simulink model "CMOS_Kernel_Memory_Sync"  (R2023b)
settings: Solver=VariableStepAuto  StartTime=0.0  StopTime=30000000  RelTol=1e-3
values from neighbouring files (symbols this model uses):
  AmountOfPixelsPerScanline = 400    [Kernel_Setup_Script.m]
  AmountOfRamBlocksScanlines = 5    [Kernel_Setup_Script.m]
  AmountOfRamBlocksScanlinesOffset = AmountOfRamBlocksScanlines - 1    (= 4)    [Kernel_Setup_Script.m]
  AmountOfScanlinePixels = 73700    [Kernel_Setup_Script.m]
  AmountOfScanlinePixelsOffset = AmountOfScanlinePixels - 1    (= 73699)    [Kernel_Setup_Script.m]
  AmountOfScanlines = 1100    [Kernel_Setup_Script.m]
  AmountOfScanlinesOffset = AmountOfScanlines - 1    (= 1099)    [Kernel_Setup_Script.m]
  AOPPK_Off = AmountOfPixelsPerScanline - 1    (= 399)    [Kernel_Setup_Script.m]
  AOPPS_Off = AmountOfPixelsPerScanline - 1    (= 399)    [Kernel_Setup_Script.m]
  FramePackOff_0 = FramePackOff_0 - ScanlineFifoCheck    [Kernel_Setup_Script.m]
  FramePackOff_1 = FramePackOff_1 - ScanlineFifoCheck    [Kernel_Setup_Script.m]
  FramePackOff_2 = FramePackOff_2 - ScanlineFifoCheck    [Kernel_Setup_Script.m]
  FramePackOff_3 = FramePackOff_3 - ScanlineFifoCheck    [Kernel_Setup_Script.m]
  FramePackOff_4 = FramePackOff_4 - ScanlineFifoCheck    [Kernel_Setup_Script.m]
  FramePackOff_5 = FramePackOff_5 - ScanlineFifoCheck    [Kernel_Setup_Script.m]
  KernelPackOff_0 = KernelPackOff_0 - KernelBitsPerRow    [Kernel_Setup_Script.m]
  KernelPackOff_1 = KernelPackOff_1 - KernelBitsPerRow    [Kernel_Setup_Script.m]
  KernelPackOff_2 = KernelPackOff_2 - KernelBitsPerRow    [Kernel_Setup_Script.m]
  KernelPackOff_3 = KernelPackOff_3 - KernelBitsPerRow    [Kernel_Setup_Script.m]
  Slice59DownTo48Top = (MsbOffset - (ScanlinePixelBitSizeController*1))    (= 59)    [Kernel_Setup_Script.m]
  Slice71DownTo60Top = (MsbOffset - (ScanlinePixelBitSizeController*0))    (= 71)    [Kernel_Setup_Script.m]
  TotalSectionsForFrames = AmountOfScanlines/AmountOfRamBlocksScanlines    (= 220)    [Kernel_Setup_Script.m]
  UltraRamRows = AmountOfPixelsPerScanline/ScanlineFifoCheck    [Kernel_Setup_Script.m]
  UltraRamRowsCeil = ceil(AmountOfPixelsPerScanline/ScanlineFifoCheck)    [Kernel_Setup_Script.m]
  UltraRamRowsKernel = AmountOfPixelsPerScanline/KernelBitsPerRow    (= 100)    [Kernel_Setup_Script.m]
  UltraRamRowsKernelCeil = ceil(AmountOfPixelsPerScanline/KernelBitsPerRow)    [Kernel_Setup_Script.m]
  UltraRamRowsMemorySectionOffset = UltraRamRowsCeil*AmountOfRamBlocksScanlines    [Kernel_Setup_Script.m]
  UltraRamRowsOffset = UltraRamRowsCeil - 1    [Kernel_Setup_Script.m]
undefined symbols (not defined in the file or in its folder): c, Down, sfvc784, Up, xck26
libraries: hdlBasic x4512, vmcUtilities x1
(part 11 of 39)

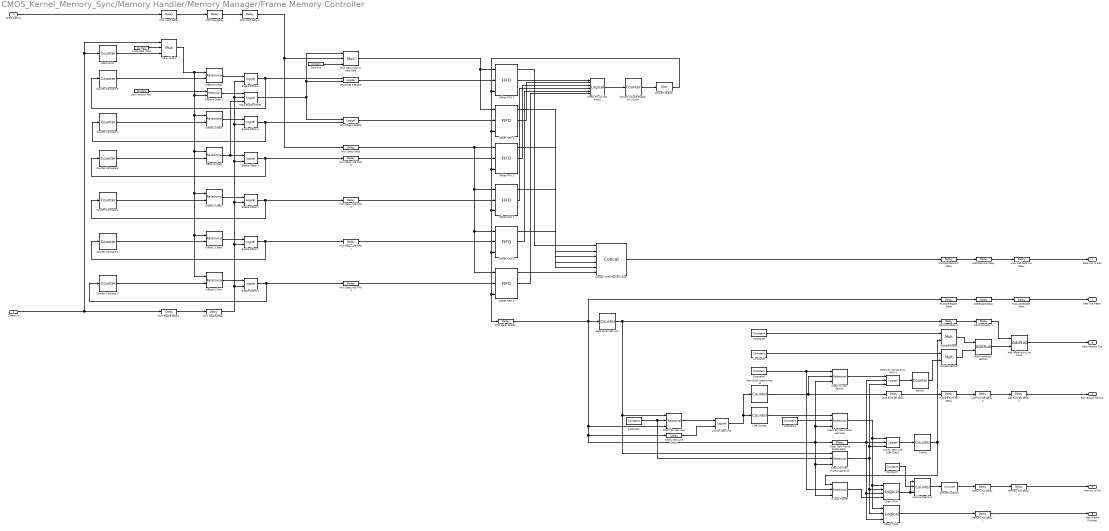
== system CMOS_Kernel_Memory_Sync/Memory Handler/Memory Manager/Frame Memory Controller ==
  12 Bit Data In : Inport
  Enable In : Inport  Port=2
  AND Input Delay : hdlBasic/Delay  rst=off  en=off  latency=1  reg_retiming=off  XmcBlockStatus=1  maskContainerNames=group1  block_type=delay  block_config=sysgen:Delay_config
  AND Input Delay2 : hdlBasic/Delay  rst=off  en=off  latency=1  reg_retiming=off  XmcBlockStatus=1  maskContainerNames=group1  block_type=delay  block_config=sysgen:Delay_config
  Add Data Out Delay : hdlBasic/Delay  rst=off  en=off  latency=1  reg_retiming=off  XmcBlockStatus=1  maskContainerNames=group1  block_type=delay  block_config=sysgen:Delay_config
  Add Enable Delay : hdlBasic/Delay  rst=off  en=off  latency=1  reg_retiming=off  XmcBlockStatus=1  maskContainerNames=group1  block_type=delay  block_config=sysgen:Delay_config
  Add Frame and Section : hdlBasic/AddSub  mode=Addition  use_carryin=off  use_carryout=off  en=off  latency=1  precision=Full  arith_type=Unsigned  n_bits=16  bin_pt=14  quantization=Truncate  overflow=Wrap  use_behavioral_HDL=off  hw_selection=Fabric  pipelined=off  XmcBlockStatus=1  maskContainerNames=tabcontainer1  block_type=addsub  block_config=sysgen:Addsub_config
  Add Line Delay 0 : hdlBasic/Delay  rst=off  en=off  latency=3  reg_retiming=off  XmcBlockStatus=1  maskContainerNames=group1  block_type=delay  block_config=sysgen:Delay_config
  Add Line Delay 1 : hdlBasic/Delay  rst=off  en=off  latency=1  reg_retiming=off  XmcBlockStatus=1  maskContainerNames=group1  block_type=delay  block_config=sysgen:Delay_config
  Add Offset with Line Count : hdlBasic/AddSub  mode=Addition  use_carryin=off  use_carryout=off  en=off  latency=1  precision=User Defined  arith_type=Unsigned  n_bits=ceil(log2(AmountOfScanlinePixels))  bin_pt=0  quantization=Truncate  overflow=Wrap  use_behavioral_HDL=off  hw_selection=Fabric  pipelined=off  XmcBlockStatus=1  maskContainerNames=tabcontainer1  block_type=addsub  block_config=sysgen:Addsub_config
  Add RAM Sel Delay 0 : hdlBasic/Delay  rst=off  en=off  latency=1  reg_retiming=off  XmcBlockStatus=1  maskContainerNames=group1  block_type=delay  block_config=sysgen:Delay_config
  Add RAM Sel Delay 1 : hdlBasic/Delay  rst=off  en=off  latency=1  reg_retiming=off  XmcBlockStatus=1  maskContainerNames=group1  block_type=delay  block_config=sysgen:Delay_config
  And RAM Sel Delay : hdlBasic/Delay  rst=off  en=off  latency=1  reg_retiming=off  XmcBlockStatus=1  maskContainerNames=group1  block_type=delay  block_config=sysgen:Delay_config
  And for New Line : hdlBasic/Logical  logical_function=AND  inputs=2  en=off  latency=1  precision=Full  arith_type=Unsigned  n_bits=16  bin_pt=0  align_bp=on  overflow=[]  quantization=[]  XmcBlockStatus=1  maskContainerNames=tabcontainer1  block_type=logical  block_config=sysgen:Logical_config
  And for New Line 1099 Check : hdlBasic/Logical  logical_function=AND  inputs=3  en=off  latency=1  precision=Full  arith_type=Unsigned  n_bits=16  bin_pt=0  align_bp=on  overflow=[]  quantization=[]  XmcBlockStatus=1  maskContainerNames=tabcontainer1  block_type=logical  block_config=sysgen:Logical_config
  Check For All Not Empty : hdlBasic/Logical  logical_function=NOR  inputs=6  en=off  latency=1  precision=Full  arith_type=Unsigned  n_bits=16  bin_pt=0  align_bp=on  overflow=[]  quantization=[]  XmcBlockStatus=1  maskContainerNames=tabcontainer1  block_type=logical  block_config=sysgen:Logical_config
  Check For New Frame Last Pixel : hdlBasic/Relational  mode=a=b  op_type=Bool  en=on  latency=1  XmcBlockStatus=1  maskContainerNames=tabcontainer1  block_type=relational  block_config=sysgen:Relational_config
  Check New Frame Enable Delay : hdlBasic/Delay  rst=off  en=off  latency=1  reg_retiming=off  XmcBlockStatus=1  maskContainerNames=group1  block_type=delay  block_config=sysgen:Delay_config
  Check New Line Delay : hdlBasic/Delay  rst=off  en=off  latency=1  reg_retiming=off  XmcBlockStatus=1  maskContainerNames=group1  block_type=delay  block_config=sysgen:Delay_config
  Check for New Frame Last Row : hdlBasic/Relational  mode=a=b  op_type=Bool  en=on  latency=1  XmcBlockStatus=1  maskContainerNames=tabcontainer1  block_type=relational  block_config=sysgen:Relational_config
  Check for last pixel on RAM 4 : hdlBasic/Logical  logical_function=AND  inputs=3  en=off  latency=1  precision=Full  arith_type=Unsigned  n_bits=16  bin_pt=0  align_bp=on  overflow=[]  quantization=[]  XmcBlockStatus=1  maskContainerNames=tabcontainer1  block_type=logical  block_config=sysgen:Logical_config
  Check for new Line : hdlBasic/Relational  mode=a=b  op_type=Bool  en=on  latency=1  XmcBlockStatus=1  maskContainerNames=tabcontainer1  block_type=relational  block_config=sysgen:Relational_config
  Check for new Section : hdlBasic/Relational  mode=a=b  op_type=Bool  en=on  latency=1  XmcBlockStatus=1  maskContainerNames=tabcontainer1  block_type=relational  block_config=sysgen:Relational_config
  Check if full : hdlBasic/Logical  logical_function=AND  inputs=4  en=off  latency=1  precision=Full  arith_type=Unsigned  n_bits=16  bin_pt=0  align_bp=on  overflow=[]  quantization=[]  XmcBlockStatus=1  maskContainerNames=tabcontainer1  block_type=logical  block_config=sysgen:Logical_config
  Check if full1 : hdlBasic/Logical  logical_function=AND  inputs=3  en=off  latency=1  precision=Full  arith_type=Unsigned  n_bits=16  bin_pt=0  align_bp=on  overflow=[]  quantization=[]  XmcBlockStatus=1  maskContainerNames=tabcontainer1  block_type=logical  block_config=sysgen:Logical_config
  Concat 72 Bit Packed Value : hdlBasic/Concat  num_inputs=ScanlineFifoCheck  XmcBlockStatus=1  maskContainerNames=group1  block_type=concat  block_config=sysgen:Concat_config
  Constant2 : hdlBasic/Constant  const=UltraRamRowsOffset  gui_display_data_type=Fixed-point  arith_type=Unsigned  n_bits=ceil(log2(UltraRamRows))  bin_pt=0  preci_type=Single  exp_width=8  frac_width=24  explicit_period=off  period=1  XmcBlockStatus=1  maskContainerNames=tabcontainer1  block_type=constant  block_config=sysgen:Constant_config
  Constant3 : hdlBasic/Constant  const=UltraRamRowsCeil  gui_display_data_type=Fixed-point  arith_type=Unsigned  n_bits=ceil(log2(UltraRamRowsCeil+1))  bin_pt=0  preci_type=Single  exp_width=8  frac_width=24  explicit_period=off  period=1  XmcBlockStatus=1  maskContainerNames=tabcontainer1  block_type=constant  block_config=sysgen:Constant_config
  Constant4 : hdlBasic/Constant  const=AmountOfScanlinesOffset  gui_display_data_type=Fixed-point  arith_type=Unsigned  n_bits=ceil(log2(AmountOfScanlines))  bin_pt=0  preci_type=Single  exp_width=8  frac_width=24  explicit_period=off  period=1  XmcBlockStatus=1  maskContainerNames=tabcontainer1  block_type=constant  block_config=sysgen:Constant_config
  Constant5 : hdlBasic/Constant  const=UltraRamRowsMemorySectionOffset  gui_display_data_type=Fixed-point  arith_type=Unsigned  n_bits=ceil(log2(UltraRamRowsMemorySectionOffset+1))  bin_pt=0  preci_type=Single  exp_width=8  frac_width=24  explicit_period=off  period=1  XmcBlockStatus=1  maskContainerNames=tabcontainer1  block_type=constant  block_config=sysgen:Constant_config
  Constant6 : hdlBasic/Constant  const=AmountOfRamBlocksScanlinesOffset  gui_display_data_type=Fixed-point  arith_type=Unsigned  n_bits=ceil(log2(AmountOfRamBlocksScanlines))  bin_pt=0  preci_type=Single  exp_width=8  frac_width=24  explicit_period=off  period=1  XmcBlockStatus=1  maskContainerNames=tabcontainer1  block_type=constant  block_config=sysgen:Constant_config
  Constant7 : hdlBasic/Constant  const=1  gui_display_data_type=Fixed-point  arith_type=Unsigned  n_bits=1  bin_pt=0  preci_type=Single  exp_width=8  frac_width=24  explicit_period=off  period=1  XmcBlockStatus=1  maskContainerNames=tabcontainer1  block_type=constant  block_config=sysgen:Constant_config
  Convert 2 Cycle Enable to 1 Cycle : hdlBasic/Counter  cnt_type=Count limited  cnt_to=2  operation=Up  start_count=0  cnt_by_val=1  arith_type=Unsigned  n_bits=2  bin_pt=0  load_pin=off  rst=off  en=on  explicit_period=Explicit  period=1  use_behavioral_HDL=off  implementation=Fabric  XmcBlockStatus=1  maskContainerNames=group1  block_type=counter  block_config=sysgen:Counter_config  block_width=531  block_height=1023
  Convert to BOOL : hdlBasic/Convert  gui_display_data_type=Boolean  arith_type=Boolean  n_bits=16  bin_pt=14  float_type=Single  exp_bits=8  fraction_bits=24  quantization=Truncate  overflow=Wrap  en=off  latency=3  pipeline=off  XmcBlockStatus=1  maskContainerNames=group2  block_type=convert  block_config=sysgen:Convert_config  block_width=595  block_height=885
  Convert to Bool : hdlBasic/Slice  nbits=1  boolean_output=on  mode=Upper Bit Location + Width  bit1=0  base1=LSB of Input  bit0=0  base0=LSB of Input  XmcBlockStatus=1  maskContainerNames=group1  block_type=slice  block_config=sysgen:Slice_config
  "Counter Compare 0  " : hdlBasic/Counter  cnt_type=Count limited  cnt_to=FramePackOff_0  operation=Up  start_count=0  cnt_by_val=6  arith_type=Unsigned  n_bits=ceil(log2(FramePackOff_0+1))  bin_pt=0  load_pin=off  rst=off  en=on  explicit_period=Explicit  period=1  use_behavioral_HDL=off  implementation=Fabric  XmcBlockStatus=1  maskContainerNames=group1  block_type=counter  block_config=sysgen:Counter_config  block_width=531  block_height=1023
  Counter Compare 1 : hdlBasic/Counter  cnt_type=Count limited  cnt_to=FramePackOff_1  operation=Up  start_count=1  cnt_by_val=6  arith_type=Unsigned  n_bits=ceil(log2(FramePackOff_1+1))  bin_pt=0  load_pin=off  rst=off  en=on  explicit_period=Explicit  period=1  use_behavioral_HDL=off  implementation=Fabric  XmcBlockStatus=1  maskContainerNames=group1  block_type=counter  block_config=sysgen:Counter_config  block_width=531  block_height=1023
  Counter Compare 2 : hdlBasic/Counter  cnt_type=Count limited  cnt_to=FramePackOff_2  operation=Up  start_count=2  cnt_by_val=6  arith_type=Unsigned  n_bits=ceil(log2(FramePackOff_2+1))  bin_pt=0  load_pin=off  rst=off  en=on  explicit_period=Explicit  period=1  use_behavioral_HDL=off  implementation=Fabric  XmcBlockStatus=1  maskContainerNames=group1  block_type=counter  block_config=sysgen:Counter_config  block_width=531  block_height=1023
  Counter Compare 3 : hdlBasic/Counter  cnt_type=Count limited  cnt_to=FramePackOff_3  operation=Up  start_count=3  cnt_by_val=6  arith_type=Unsigned  n_bits=ceil(log2(FramePackOff_3+1))  bin_pt=0  load_pin=off  rst=off  en=on  explicit_period=Explicit  period=1  use_behavioral_HDL=off  implementation=Fabric  XmcBlockStatus=1  maskContainerNames=group1  block_type=counter  block_config=sysgen:Counter_config  block_width=531  block_height=1023
  Counter Compare 4 : hdlBasic/Counter  cnt_type=Count limited  cnt_to=FramePackOff_4  operation=Up  start_count=4  cnt_by_val=6  arith_type=Unsigned  n_bits=ceil(log2(FramePackOff_4+1))  bin_pt=0  load_pin=off  rst=off  en=on  explicit_period=Explicit  period=1  use_behavioral_HDL=off  implementation=Fabric  XmcBlockStatus=1  maskContainerNames=group1  block_type=counter  block_config=sysgen:Counter_config  block_width=531  block_height=1023
  Counter Compare 5 : hdlBasic/Counter  cnt_type=Count limited  cnt_to=FramePackOff_5  operation=Up  start_count=5  cnt_by_val=6  arith_type=Unsigned  n_bits=ceil(log2(FramePackOff_5+1))  bin_pt=0  load_pin=off  rst=off  en=on  explicit_period=Explicit  period=1  use_behavioral_HDL=off  implementation=Fabric  XmcBlockStatus=1  maskContainerNames=group1  block_type=counter  block_config=sysgen:Counter_config  block_width=531  block_height=1023
  Data Points : hdlBasic/Counter  cnt_type=Count limited  cnt_to=AOPPS_Off  operation=Up  start_count=0  cnt_by_val=1  arith_type=Unsigned  n_bits=ceil(log2(AOPPS_Off+1))  bin_pt=0  load_pin=off  rst=off  en=on  explicit_period=Explicit  period=1  use_behavioral_HDL=off  implementation=Fabric  XmcBlockStatus=1  maskContainerNames=group1  block_type=counter  block_config=sysgen:Counter_config  block_width=531  block_height=1023
  Data Points Per Line : hdlBasic/Counter  cnt_type=Count limited  cnt_to=UltraRamRowsOffset  operation=Up  start_count=0  cnt_by_val=1  arith_type=Unsigned  n_bits=ceil(log2(UltraRamRowsOffset + 1))  bin_pt=0  load_pin=off  rst=off  en=on  explicit_period=Explicit  period=1  use_behavioral_HDL=off  implementation=Fabric  XmcBlockStatus=1  maskContainerNames=group1  block_type=counter  block_config=sysgen:Counter_config  block_width=531  block_height=1023
  Enable Offset {0..5} (6 alike) : hdlBasic/Logical  logical_function=AND  inputs=2  en=off  latency=1  precision=Full  arith_type=Unsigned  n_bits=16  bin_pt=0  align_bp=on  overflow=[]  quantization=[]  XmcBlockStatus=1  maskContainerNames=tabcontainer1  block_type=logical  block_config=sysgen:Logical_config
  FIFO Delay Enable : hdlBasic/Delay  rst=off  en=off  latency=1  reg_retiming=off  XmcBlockStatus=1  maskContainerNames=group1  block_type=delay  block_config=sysgen:Delay_config
  Final Add Data Out Delay : hdlBasic/Delay  rst=off  en=off  latency=1  reg_retiming=off  XmcBlockStatus=1  maskContainerNames=group1  block_type=delay  block_config=sysgen:Delay_config
  Final Add Enable Delay : hdlBasic/Delay  rst=off  en=off  latency=1  reg_retiming=off  XmcBlockStatus=1  maskContainerNames=group1  block_type=delay  block_config=sysgen:Delay_config
  Frame : hdlBasic/Counter  cnt_type=Count limited  cnt_to=AmountOfRamBlocksScanlinesOffset  operation=Up  start_count=0  cnt_by_val=1  arith_type=Unsigned  n_bits=ceil(log2(AmountOfRamBlocksScanlines+1))  bin_pt=0  load_pin=off  rst=off  en=on  explicit_period=Explicit  period=1  use_behavioral_HDL=off  implementation=Fabric  XmcBlockStatus=1  maskContainerNames=group1  block_type=counter  block_config=sysgen:Counter_config  block_width=531  block_height=1023
  Hold Up Read Out : hdlBasic/Counter  cnt_type=Free running  cnt_to=1  operation=Up  start_count=0  cnt_by_val=1  arith_type=Unsigned  n_bits=1  bin_pt=0  load_pin=on  rst=off  en=on  explicit_period=Explicit  period=1  use_behavioral_HDL=off  implementation=Fabric  XmcBlockStatus=1  maskContainerNames=group1  block_type=counter  block_config=sysgen:Counter_config  block_width=531  block_height=1023
  Impossible Value : hdlBasic/Constant  const=AOPPS_Off + 1  gui_display_data_type=Fixed-point  arith_type=Unsigned  n_bits=ceil(log2(AmountOfPixelsPerScanline + 1))  bin_pt=0  preci_type=Single  exp_width=8  frac_width=24  explicit_period=off  period=1  XmcBlockStatus=1  maskContainerNames=tabcontainer1  block_type=constant  block_config=sysgen:Constant_config
  Is Last Frame? : hdlBasic/Relational  mode=a=b  op_type=Bool  en=on  latency=1  XmcBlockStatus=1  maskContainerNames=tabcontainer1  block_type=relational  block_config=sysgen:Relational_config
  Last Value to Pack : hdlBasic/Constant  const=AOPPS_Off  gui_display_data_type=Fixed-point  arith_type=Unsigned  n_bits=ceil(log2(AmountOfPixelsPerScanline))  bin_pt=0  preci_type=Single  exp_width=8  frac_width=24  explicit_period=off  period=1  XmcBlockStatus=1  maskContainerNames=tabcontainer1  block_type=constant  block_config=sysgen:Constant_config
  Line Counter : hdlBasic/Counter  cnt_type=Count limited  cnt_to=AmountOfScanlinesOffset  operation=Up  start_count=0  cnt_by_val=1  arith_type=Unsigned  n_bits=ceil(log2(AmountOfScanlines))  bin_pt=0  load_pin=off  rst=off  en=on  explicit_period=Explicit  period=1  use_behavioral_HDL=off  implementation=Fabric  XmcBlockStatus=1  maskContainerNames=group1  block_type=counter  block_config=sysgen:Counter_config  block_width=531  block_height=1023
  MUX Delay Input : hdlBasic/Delay  rst=off  en=off  latency=1  reg_retiming=off  XmcBlockStatus=1  maskContainerNames=group1  block_type=delay  block_config=sysgen:Delay_config
  MUX Delay WE FIFO {0..3} (4 alike) : hdlBasic/Delay  rst=off  en=off  latency=1  reg_retiming=off  XmcBlockStatus=1  maskContainerNames=group1  block_type=delay  block_config=sysgen:Delay_config
  MUX Enable Delay : hdlBasic/Delay  rst=off  en=off  latency=1  reg_retiming=off  XmcBlockStatus=1  maskContainerNames=group1  block_type=delay  block_config=sysgen:Delay_config
  MUX Enable Delay1 : hdlBasic/Delay  rst=off  en=off  latency=1  reg_retiming=off  XmcBlockStatus=1  maskContainerNames=group1  block_type=delay  block_config=sysgen:Delay_config
  MUX Input Delay : hdlBasic/Delay  rst=off  en=off  latency=1  reg_retiming=off  XmcBlockStatus=1  maskContainerNames=group1  block_type=delay  block_config=sysgen:Delay_config
  MUX Zero Value or Input Data : hdlBasic/Mux  inputs=2  en=off  latency=1  precision=Full  arith_type=Unsigned  n_bits=16  bin_pt=14  quantization=Truncate  overflow=Wrap  XmcBlockStatus=1  maskContainerNames=tabcontainer1  block_type=mux  block_config=sysgen:Mux_config
  Mass Enable Offset : hdlBasic/Logical  logical_function=AND  inputs=3  en=off  latency=1  precision=Full  arith_type=Unsigned  n_bits=16  bin_pt=0  align_bp=on  overflow=[]  quantization=[]  XmcBlockStatus=1  maskContainerNames=tabcontainer1  block_type=logical  block_config=sysgen:Logical_config
  Memory Full Delay 0 : hdlBasic/Delay  rst=off  en=off  latency=1  reg_retiming=off  XmcBlockStatus=1  maskContainerNames=group1  block_type=delay  block_config=sysgen:Delay_config
  Memory Full Delay 1 : hdlBasic/Delay  rst=off  en=off  latency=1  reg_retiming=off  XmcBlockStatus=1  maskContainerNames=group1  block_type=delay  block_config=sysgen:Delay_config
  Memory Full Delay 2 : hdlBasic/Delay  rst=off  en=off  latency=6  reg_retiming=off  XmcBlockStatus=1  maskContainerNames=group1  block_type=delay  block_config=sysgen:Delay_config
  Multiple Data Out Delay : hdlBasic/Delay  rst=off  en=off  latency=3  reg_retiming=off  XmcBlockStatus=1  maskContainerNames=group1  block_type=delay  block_config=sysgen:Delay_config
  Multiple Enable Delay : hdlBasic/Delay  rst=off  en=off  latency=3  reg_retiming=off  XmcBlockStatus=1  maskContainerNames=group1  block_type=delay  block_config=sysgen:Delay_config
  Multiple Frame : hdlBasic/Mult  precision=Full  arith_type="Signed  (2's comp)"  n_bits=16  bin_pt=14  quantization=Truncate  overflow=Wrap  en=off  latency=3  use_behavioral_HDL=off  opt=Speed  use_embedded=on  optimum_pipeline=off  pipeline=on  use_rpm=on  placement_style=Triangular  XmcBlockStatus=1  maskContainerNames=group1  block_type=mult  block_config=sysgen:Mult_config  block_width=598  block_height=876
  Multiple RAM Sel Delay : hdlBasic/Delay  rst=off  en=off  latency=3  reg_retiming=off  XmcBlockStatus=1  maskContainerNames=group1  block_type=delay  block_config=sysgen:Delay_config
  Multiple Section : hdlBasic/Mult  precision=Full  arith_type="Signed  (2's comp)"  n_bits=16  bin_pt=14  quantization=Truncate  overflow=Wrap  en=off  latency=3  use_behavioral_HDL=off  opt=Speed  use_embedded=on  optimum_pipeline=off  pipeline=on  use_rpm=on  placement_style=Triangular  XmcBlockStatus=1  maskContainerNames=group1  block_type=mult  block_config=sysgen:Mult_config  block_width=598  block_height=876
  OR Offset 4 Enable : hdlBasic/Logical  logical_function=OR  inputs=2  en=off  latency=1  precision=Full  arith_type=Unsigned  n_bits=16  bin_pt=0  align_bp=on  overflow=[]  quantization=[]  XmcBlockStatus=1  maskContainerNames=tabcontainer1  block_type=logical  block_config=sysgen:Logical_config
  OR Offset 5 Enable : hdlBasic/Logical  logical_function=OR  inputs=2  en=off  latency=1  precision=Full  arith_type=Unsigned  n_bits=16  bin_pt=0  align_bp=on  overflow=[]  quantization=[]  XmcBlockStatus=1  maskContainerNames=tabcontainer1  block_type=logical  block_config=sysgen:Logical_config
  Offset 0 Check : hdlBasic/Relational  mode=a=b  op_type=Bool  en=off  latency=1  XmcBlockStatus=1  maskContainerNames=tabcontainer1  block_type=relational  block_config=sysgen:Relational_config
  Offset 1 Check : hdlBasic/Relational  mode=a=b  op_type=Bool  en=off  latency=1  XmcBlockStatus=1  maskContainerNames=tabcontainer1  block_type=relational  block_config=sysgen:Relational_config
  Offset 2 Check : hdlBasic/Relational  mode=a=b  op_type=Bool  en=off  latency=1  XmcBlockStatus=1  maskContainerNames=tabcontainer1  block_type=relational  block_config=sysgen:Relational_config
  Offset 3 Check : hdlBasic/Relational  mode=a=b  op_type=Bool  en=off  latency=1  XmcBlockStatus=1  maskContainerNames=tabcontainer1  block_type=relational  block_config=sysgen:Relational_config
  Offset 4 Check : hdlBasic/Relational  mode=a=b  op_type=Bool  en=off  latency=1  XmcBlockStatus=1  maskContainerNames=tabcontainer1  block_type=relational  block_config=sysgen:Relational_config
  Offset 4 Check1 : hdlBasic/Relational  mode=a=b  op_type=Bool  en=off  latency=1  XmcBlockStatus=1  maskContainerNames=tabcontainer1  block_type=relational  block_config=sysgen:Relational_config
  Offset 5 Check : hdlBasic/Relational  mode=a=b  op_type=Bool  en=off  latency=1  XmcBlockStatus=1  maskContainerNames=tabcontainer1  block_type=relational  block_config=sysgen:Relational_config
  Offset FIFO {0..5} (6 alike) : hdlBasic/FIFO  mem_type=Block RAM  performance_options=Standard_FIFO  embedded_registers=off  depth=16  use_asym_data_widths=off  asym_read_width=32  percent_nbits=4  rst=off  rst_latency=2  en=off  use_dcount=off  use_percent_full_port=off  use_almost_empty=off  almost_empty_thresh=2  use_almost_full=off  use_rd_rst_busy=off  use_wr_rst_busy=off  almost_full_thresh=14  almost_empty_offset=[]  almost_full_offset=[]  explicit_period=off  period=[]  store_only_valid=[]  init_zero=[]  simulation_type=fast_sim  XmcBlockStatus=1  maskContainerNames=tabcontainer1  block_type=fifo  block_config=sysgen:FIFO_config  block_width=538  block_height=997
      settings: infoedit=[]
  Ram Block Determination : hdlBasic/Counter  cnt_type=Count limited  cnt_to=AmountOfRamBlocksScanlinesOffset  operation=Up  start_count=0  cnt_by_val=1  arith_type=Unsigned  n_bits=ceil(log2(AmountOfRamBlocksScanlines))  bin_pt=0  load_pin=off  rst=off  en=on  explicit_period=Explicit  period=1  use_behavioral_HDL=off  implementation=Fabric  XmcBlockStatus=1  maskContainerNames=group1  block_type=counter  block_config=sysgen:Counter_config  block_width=531  block_height=1023
  Section : hdlBasic/Counter  cnt_type=Count limited  cnt_to=TotalSectionsForFramesOffset  operation=Up  start_count=0  cnt_by_val=1  arith_type=Unsigned  n_bits=ceil(log2(TotalSectionsForFrames))  bin_pt=0  load_pin=off  rst=off  en=on  explicit_period=Explicit  period=1  use_behavioral_HDL=off  implementation=Fabric  XmcBlockStatus=1  maskContainerNames=group1  block_type=counter  block_config=sysgen:Counter_config  block_width=531  block_height=1023
  Zero Out : hdlBasic/Constant  const=0  gui_display_data_type=Fixed-point  arith_type=Unsigned  n_bits=12  bin_pt=0  preci_type=Single  exp_width=8  frac_width=24  explicit_period=off  period=1  XmcBlockStatus=1  maskContainerNames=tabcontainer1  block_type=constant  block_config=sysgen:Constant_config
  Zero Value1 : hdlBasic/Mux  inputs=2  en=off  latency=1  precision=Full  arith_type=Unsigned  n_bits=16  bin_pt=14  quantization=Truncate  overflow=Wrap  XmcBlockStatus=1  maskContainerNames=tabcontainer1  block_type=mux  block_config=sysgen:Mux_config
  Data Out 72 Bits : Outport
  Data Out Ready : Outport  Port=2
  Data Address Out : Outport  Port=3
  Ram Bloack Sel Out : Outport  Port=4
  Memory Is Full : Outport  Port=5
  New Frame Finished : Outport  Port=6
  wires:
  FIFO Delay Enable/1 -> Multiple Enable Delay/1, Check for new Line/3, Check New Line Delay/1, Is Last Frame?/3, Check For New Frame Last Pixel/3, Check for new Section/3, Check for New Frame Last Row/3, Check New Frame Enable Delay/1, Data Points Per Line/1
  Offset FIFO 4/1 -> Concat 72 Bit Packed Value/2
  Constant4/1 -> Check for New Frame Last Row/2
  Add RAM Sel Delay 1/1 -> Ram Bloack Sel Out/1
  Offset FIFO 4/2 -> Check For All Not Empty/2
  And for New Line 1099 Check/1 -> Frame/1
  Add Line Delay 0/1 -> Add Line Delay 1/1
  Offset FIFO 3/2 -> Check For All Not Empty/3
  Offset FIFO 2/1 -> Concat 72 Bit Packed Value/4
  Constant5/1 -> Multiple Section/1
  Convert to Bool/1 -> FIFO Delay Enable/1, Offset FIFO 0/3, Offset FIFO 1/3, Offset FIFO 2/3, Offset FIFO 3/3, Offset FIFO 4/3, Offset FIFO 5/3
  Add RAM Sel Delay 0/1 -> Add RAM Sel Delay 1/1
  Constant3/1 -> Multiple Frame/1
  Check New Line Delay/1 -> And for New Line/2
  Offset FIFO 0/1 -> Concat 72 Bit Packed Value/6
  Constant2/1 -> Check For New Frame Last Pixel/2, Check for new Line/2
  Zero Value1/1 -> Offset 4 Check1/2, Offset 0 Check/1, Offset 1 Check/1, Offset 2 Check/1, Offset 3 Check/1, Offset 4 Check/1, Offset 5 Check/1
  Check For New Frame Last Pixel/1 -> Check if full1/2, Check if full/2, Check for last pixel on RAM 4/3, And for New Line 1099 Check/3
  Frame/1 -> Is Last Frame?/1, Multiple Frame/2
  Offset FIFO 0/2 -> Check For All Not Empty/6
  Constant6/1 -> Check for new Section/1, Is Last Frame?/2
  Check for New Frame Last Row/1 -> Check if full1/1, Check if full/1, And for New Line 1099 Check/1
  Add Enable Delay/1 -> Final Add Enable Delay/1
  Multiple Frame/1 -> Add Frame and Section/1
  Data Points Per Line/1 -> Check for new Line/1, Check For New Frame Last Pixel/1, Add Line Delay 0/1
  Check For All Not Empty/1 -> Convert 2 Cycle Enable to 1 Cycle/1
  Add Data Out Delay/1 -> Final Add Data Out Delay/1
  Multiple RAM Sel Delay/1 -> Add RAM Sel Delay 0/1
  Offset FIFO 2/2 -> Check For All Not Empty/4
  Multiple Enable Delay/1 -> Add Enable Delay/1
  Check for new Line/1 -> And for New Line/1
  Check New Frame Enable Delay/1 -> And for New Line 1099 Check/2, Check if full1/3, Check if full/3, Check for last pixel on RAM 4/2
  Offset FIFO 1/2 -> Check For All Not Empty/5
  Ram Block Determination/1 -> And RAM Sel Delay/1, Check for new Section/2
  Offset FIFO 1/1 -> Concat 72 Bit Packed Value/5
  Line Counter/1 -> Check for New Frame Last Row/1
  Offset FIFO 5/2 -> Check For All Not Empty/1
  Offset FIFO 3/1 -> Concat 72 Bit Packed Value/3
  And for New Line/1 -> Ram Block Determination/1, Line Counter/1
  Convert 2 Cycle Enable to 1 Cycle/1 -> Convert to Bool/1
  Add Frame and Section/1 -> Add Offset with Line Count/2
  Concat 72 Bit Packed Value/1 -> Multiple Data Out Delay/1
  Offset FIFO 5/1 -> Concat 72 Bit Packed Value/1
  And RAM Sel Delay/1 -> Multiple RAM Sel Delay/1
  Last Value to Pack/1 -> Offset 4 Check1/1
  Check for new Section/1 -> Check for last pixel on RAM 4/1
  Section/1 -> Multiple Section/2
  Multiple Section/1 -> Add Frame and Section/2
  Add Line Delay 1/1 -> Add Offset with Line Count/1
  Multiple Data Out Delay/1 -> Add Data Out Delay/1
  Check for last pixel on RAM 4/1 -> Section/1
  Final Add Data Out Delay/1 -> Data Out 72 Bits/1
  Final Add Enable Delay/1 -> Data Out Ready/1
  Add Offset with Line Count/1 -> Data Address Out/1
  Memory Full Delay 1/1 -> Memory Is Full/1
  Is Last Frame?/1 -> Check if full/4
  Check if full/1 -> Hold Up Read Out/1, Hold Up Read Out/3
  Hold Up Read Out/1 -> Convert to BOOL/1
  Convert to BOOL/1 -> Memory Full Delay 0/1
  Constant7/1 -> Hold Up Read Out/2
  Memory Full Delay 0/1 -> Memory Full Delay 1/1
  Memory Full Delay 2/1 -> New Frame Finished/1
  Check if full1/1 -> Memory Full Delay 2/1
  Zero Out/1 -> MUX Zero Value or Input Data/3
  Data Points/1 -> Zero Value1/3
  Offset 0 Check/1 -> Enable Offset 0/1
  Offset 4 Check1/1 -> Mass Enable Offset/1
  Offset 5 Check/1 -> Enable Offset 5/1
  Offset 4 Check/1 -> Enable Offset 4/1
  Offset 3 Check/1 -> Mass Enable Offset/3, Enable Offset 3/1
  Offset 2 Check/1 -> Enable Offset 2/1
  Offset 1 Check/1 -> Enable Offset 1/1
  Enable In/1 -> Zero Value1/1, Data Points/1, MUX Enable Delay1/1
  Impossible Value/1 -> Zero Value1/2
  "Counter Compare 0  "/1 -> Offset 0 Check/2
  Counter Compare 1/1 -> Offset 1 Check/2
  Counter Compare 2/1 -> Offset 2 Check/2
  Counter Compare 3/1 -> Offset 3 Check/2
  Counter Compare 4/1 -> Offset 4 Check/2
  Counter Compare 5/1 -> Offset 5 Check/2
  OR Offset 4 Enable/1 -> Offset FIFO 4/2
  OR Offset 5 Enable/1 -> Offset FIFO 5/2
  MUX Delay WE FIFO 3/1 -> Offset FIFO 3/2
  MUX Delay WE FIFO 2/1 -> Offset FIFO 2/2
  MUX Delay WE FIFO 1/1 -> Offset FIFO 1/2
  MUX Delay WE FIFO 0/1 -> Offset FIFO 0/2
  Enable Offset 0/1 -> MUX Delay WE FIFO 0/1, "Counter Compare 0  "/1
  Enable Offset 1/1 -> MUX Delay WE FIFO 1/1, Counter Compare 1/1
  Enable Offset 2/1 -> MUX Delay WE FIFO 2/1, Counter Compare 2/1
  Enable Offset 3/1 -> MUX Delay WE FIFO 3/1, Counter Compare 3/1
  AND Input Delay/1 -> AND Input Delay2/1
  Enable Offset 4/1 -> OR Offset 4 Enable/2, Counter Compare 4/1
  Enable Offset 5/1 -> OR Offset 5 Enable/1, Counter Compare 5/1
  MUX Delay Input/1 -> Offset FIFO 0/1, Offset FIFO 1/1, Offset FIFO 2/1, Offset FIFO 3/1
  MUX Zero Value or Input Data/1 -> Offset FIFO 5/1, Offset FIFO 4/1
  Mass Enable Offset/1 -> OR Offset 4 Enable/1, OR Offset 5 Enable/2, MUX Zero Value or Input Data/1
  MUX Enable Delay/1 -> Enable Offset 0/2, Enable Offset 1/2, Enable Offset 2/2, Enable Offset 3/2, Enable Offset 5/2, Mass Enable Offset/2, Enable Offset 4/2
  MUX Input Delay/1 -> AND Input Delay/1
  AND Input Delay2/1 -> MUX Delay Input/1, MUX Zero Value or Input Data/2
  MUX Enable Delay1/1 -> MUX Enable Delay/1
  12 Bit Data In/1 -> MUX Input Delay/1
